simulink model "Refined_Model"  (R2016a)
settings: Solver=VariableStepAuto  StartTime=0.0  StopTime=20  RelTol=1e-3
values from neighbouring files (symbols this model uses):
  b = 0.000931    [Model.m]    (also in Projekt_disturbance.m; Rlocus.m = 3.5077e-06)
  J = 0.3    [Model.m]    (also in Projekt_disturbance.m = 0.00567; Rlocus.m = 3.2284e-06)
  Kb = 0.509    [Model.m]    (also in Projekt_disturbance.m)
  Km = 0.509    [Model.m]    (also in Projekt_disturbance.m)
  Ra = 7.101    [Model.m]    (also in Projekt_disturbance.m)
settings Model: Creator=Kristian  LastModifiedBy=Kristian

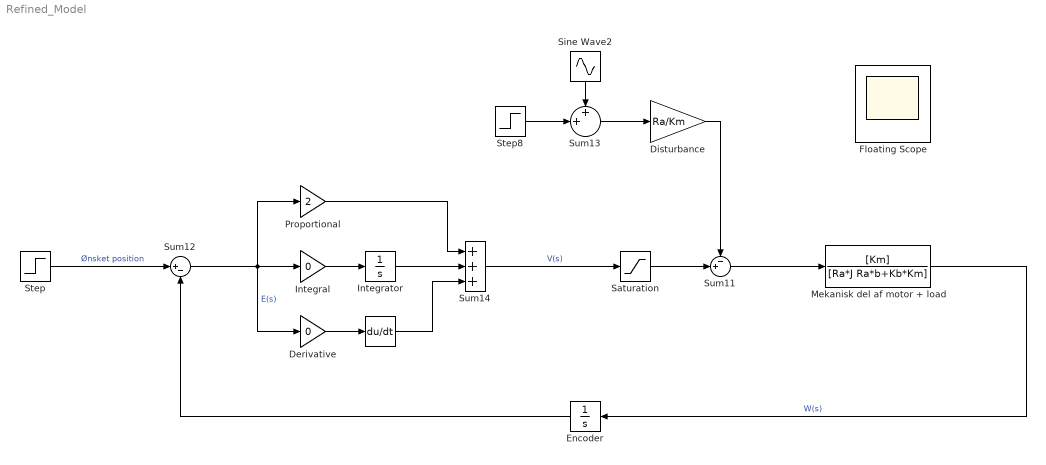
== system Refined_Model ==
  " " : Derivative
  Derivative : Gain  Gain=0  OutMin=-5  OutMax=5
  Disturbance : Gain  Gain=Ra/Km  OutMin=-5  OutMax=5
  Encoder : Integrator
  Floating Scope : Scope
      settings: Floating=on
  Integral : Gain  Gain=0  OutMin=-5  OutMax=5
  Integrator : Integrator
  Mekanisk del af motor + load : TransferFcn  Numerator=[Km]  Denominator=[Ra*J Ra*b+Kb*Km]
  Proportional : Gain  Gain=2  OutMin=-5  OutMax=5
  Saturation : Saturate  UpperLimit=5  LowerLimit=-5
  Sine Wave2 : Sin  Amplitude=0  Frequency=0.1  SampleTime=0
  Step : Step  SampleTime=0
  Step8 : Step  Time=10  After=0  SampleTime=0
  Sum11 : Sum  Inputs=-+|
  Sum12 : Sum  Inputs=|+-
  Sum13 : Sum  Inputs=++|
  Sum14 : Sum  Inputs=+++
  wires:
  Sum11/1 -> Mekanisk del af motor + load/1
  Mekanisk del af motor + load/1 -> Encoder/1  "W(s)"
  Sum12/1 -> Derivative/1, Integral/1, Proportional/1  "E(s)"
  Step/1 -> Sum12/1  "Ønsket position"
  Step8/1 -> Sum13/2
  Sine Wave2/1 -> Sum13/1
  Proportional/1 -> Sum14/1
  Integral/1 -> Integrator/1
  Integrator/1 -> Sum14/2
  Derivative/1 -> " "/1
  " "/1 -> Sum14/3
  Encoder/1 -> Sum12/2
  Sum13/1 -> Disturbance/1
  Disturbance/1 -> Sum11/1
  Sum14/1 -> Saturation/1  "V(s)"
  Saturation/1 -> Sum11/2
